simulink model "dc_motor_speed_with_compensators"  (R2021b)
settings: Solver=VariableStepAuto  StartTime=0.0  StopTime=10.0  RelTol=1e-3
values from neighbouring files (symbols this model uses):
  b = 0.1    [Lag_Lead_PI_PD_PID_and_Lag_Lead_with_the_DC_motor_plant.m]    (also in dc_motor_parameters.m; dc_motor_with_compensators_parameters.m; simscape_dc_motor.m)
  J = 0.01    [Lag_Lead_PI_PD_PID_and_Lag_Lead_with_the_DC_motor_plant.m]    (also in dc_motor_parameters.m; dc_motor_with_compensators_parameters.m; simscape_dc_motor.m)
  K = 0.01    [Lag_Lead_PI_PD_PID_and_Lag_Lead_with_the_DC_motor_plant.m]    (also in MASSDAMPERANALYSIS.m = 2; compensator_example.m = 1; compensator_example2.m = 1; dc_motor_parameters.m)
  L = minreal(C*P)    [Lag_Lead_PI_PD_PID_and_Lag_Lead_with_the_DC_motor_plant.m]    (also in dc_motor_parameters.m = 0.5; dc_motor_with_compensators_parameters.m = 0.5; simscape_dc_motor.m = 0.5)
  R = 1    [Lag_Lead_PI_PD_PID_and_Lag_Lead_with_the_DC_motor_plant.m]    (also in dc_motor_parameters.m; dc_motor_with_compensators_parameters.m; simscape_dc_motor.m)
settings Model: Creator=Joshua  LastModifiedBy=Joshua

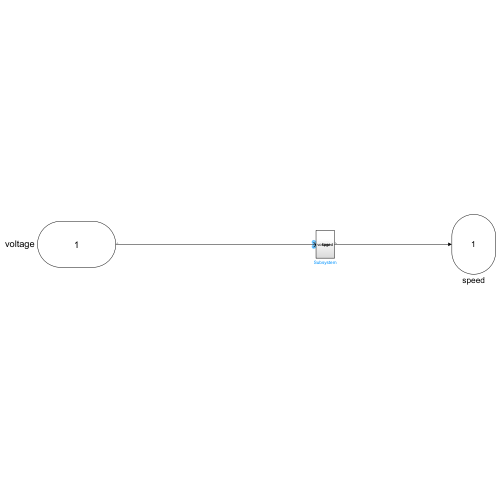
[thumbnail: Simulink's stored preview of the top-level diagram]
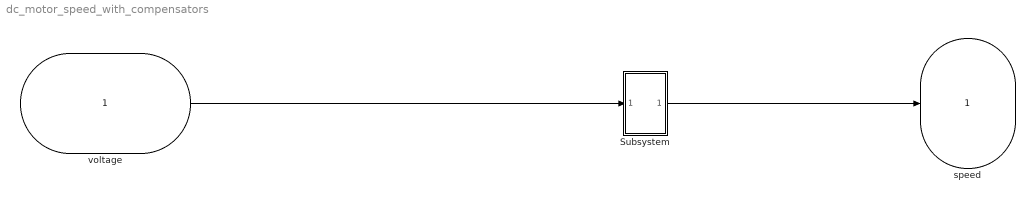
== system dc_motor_speed_with_compensators ==
  voltage : Inport
  Subsystem : Subsystem
  speed : Outport
  wires:
  voltage/1 -> Subsystem/1(voltage)
  Subsystem/1(speed) -> speed/1

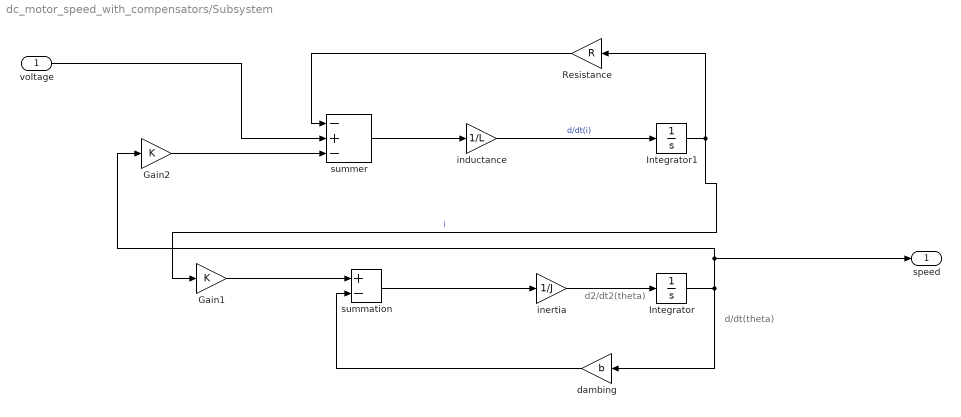
== system dc_motor_speed_with_compensators/Subsystem ==
  note: d/dt(theta)
  note: d2/dt2(theta)
  voltage : Inport
  Gain1 : Gain  Gain=K
  Gain2 : Gain  Gain=K
  Integrator : Integrator
  Integrator1 : Integrator
  Resistance : Gain  Gain=R
  dambing : Gain  Gain=b
  inductance : Gain  Gain=1/L
  inertia : Gain  Gain=1/J
  summation : Sum  Inputs=+-
  summer : Sum  Inputs=-+-
  speed : Outport
  wires:
  inductance/1 -> Integrator1/1  "d/dt(i)"
  Integrator1/1 -> Gain1/1, Resistance/1  "i"
  summer/1 -> inductance/1
  summation/1 -> inertia/1
  dambing/1 -> summation/2
  Gain1/1 -> summation/1
  Integrator/1 -> speed/1, Gain2/1, dambing/1
  voltage/1 -> summer/2
  inertia/1 -> Integrator/1
  Resistance/1 -> summer/1
  Gain2/1 -> summer/3
